simulink model "AUV_Multi_MPC"  (R2023a)
settings: Solver=ode23t  StartTime=0.0  StopTime=300  MaxStep=0.01  RelTol=1e-3  EnableMultiTasking=on
PreLoadFcn:
  | AUV_VehicleParameters;
  | Vehicle.Body.markeropacity = 0;
InitFcn:
  | %% ========================= SAMPLE TIME =========================
  | Ts = 0.1;
  | %% ========================= MPC: SURGE X =========================
  | nx = 1; nu = 1; ny = 1;
  | 
  | A = 0.9; B = 0.1; C = 1; D = 0;
  | plant = ss(A, B, C, D, Ts);
  | mpc1 = mpc(plant, Ts);
  | 
  | % Cấu hình như bình thường
  | mpc1.PredictionHorizon = 10;
  | mpc1.ControlHorizon = 2;
  | 
  | mpc1.Weights.OV = 7.5; % đủ mạnh để bám
  | mpc1.Weights.MV = 0.08; % cho dùng lực nhiều hơn
  | mpc1.Weights.MVRate = 0.25; % vừa mượt vừa linh hoạt
  | mpc1.MV.Min = -40;
  | mpc1.MV.Max = 40;
  | mpc1.OV.Min = 0;
  | mpc1.OV.Max = 2;
  | 
  | % Ràng buộc về thay đổi lực
  | mpc1.MV.RateMin = -12.5;
  | mpc1.MV.RateMax = 12.5;
  | %% ========================= MPC OUTER LOOP FOR DEPTH (Z) =========================
  | % ===== Baseline outer MPC for depth =====
  | u0 = 1.2;
  | 
  | A = 1;
  | B = -Ts*u0;
  | C = 1;
  | D = 0;
  | 
  | plant_z = ss(A,B,C,D,Ts);
  | 
  | mpc_z = mpc(plant_z,Ts);
  | mpc_z.PredictionHorizon = 10;
  | mpc_z.ControlHorizon    = 2;
  | 
  | mpc_z.Weights.OV     = 12;
  | mpc_z.Weights.MV     = 0.01;
  | mpc_z.Weights.MVRate = 0.1;
  | 
  | theta_ref_max = deg2rad(18);
  | mpc_z.MV.Min = -theta_ref_max;
  | mpc_z.MV.Max =  theta_ref_max;
  | 
  | mpc_z.MV.RateMin = -deg2rad(4);
  | mpc_z.MV.RateMax =  deg2rad(4);
  | 
  | 
  | %% ========================= MPC OUTER LOOP FOR HEADING =========================
  | A = 1;
  | B = Ts;
  | C = 1;
  | D = 0;
  | 
  | plant_psi = ss(A,B,C,D,Ts);
  | mpc_psi = mpc(plant_psi,Ts);
  | 
  | ... (+13 lines)
StopFcn:
  | try
  |     S = out;
  | 
  |     % ===============================
  |     % CHỌN HỆ QUY CHIẾU
  |     % ===============================
  |     USE_UP = true;   % true = ENU (Up), false = NED (Down)
  | 
  |     % ===============================
  |     % AUV position (NED gốc)
  |     % ===============================
  |     P  = squeeze(S.auv_position.signals.values);   % [Xn Ye Zd]
  |     tP = S.auv_position.time(:);
  | 
  |     Xn = P(:,1);   % North
  |     Ye = P(:,2);   % East
  |     Zd = P(:,3);   % Down (+)
  | 
  |     % ===============================
  |     % Reference vector
  |     % ===============================
  |     R = squeeze(S.auv_reference.signals.values);  % [V D psi]
  |     t = S.auv_reference.time(:);
  | 
  |     V   = R(:,1);      % speed
  |     D   = R(:,2);      % depth (Down +)
  |     psi = R(:,3);      % heading (rad)
  | 
  |     % ===============================
  |     % Reconstruct reference trajectory (NED)
  |     % ===============================
  |     Xr = Xn(1) + cumtrapz(t, V .* cos(psi));   % North
  |     Yr = Ye(1) + cumtrapz(t, V .* sin(psi));   % East
  |     Zr_down = Zd(1) + (D - D(1));              % Down (+)
  | 
  |     % ===============================
  |     % CHUYỂN HỆ (nếu cần)
  |     % ===============================
  |     if USE_UP
  |         Za  = -Zd;        % Up
  |         Zr  = -Zr_down;   % Up
  |         zlbl = 'Z (Up, m)';
  |     else
  |         Za  = Zd;         % Down
  |         Zr  = Zr_down;
  |         zlbl = 'Z (Down, m)';
  |     end
  | 
  |     % ===============================
  |     % Plot
  |     % ===============================
  |     f = figure(2); clf(f);
  |     set(f,'Name','AUV vs Reference','NumberTitle','off');
  | 
  |     ax = gca;
  |     ax.SortMethod = 'childorder';
  | 
  |     hRef   = plot3(Xr, Yr, Zr, '--', ...
  |                    'Color',[0.6 0.6 0.6], 'LineWidth',1.2);
  |     hold on
  | ... (+24 lines)
model workspace: external: MATLAB File AUV_DataFile_ORIG.m (data not in the file)
undefined symbols (not defined in the file): Environment, Multibody, Newton, Raphson, smiData, X, x, Y, y, Z
libraries: sm_lib x3123, nesl_utility x51, sharedutil x8, simulink x6, AUVCustomPrimitives_Lib x4, mpclib x3, fuzblock x2, instrumentseriallib x2, shared6dof x1, slpidlib x1, aerolibasang x1, aerolibadyn x1
(part 2 of 72)

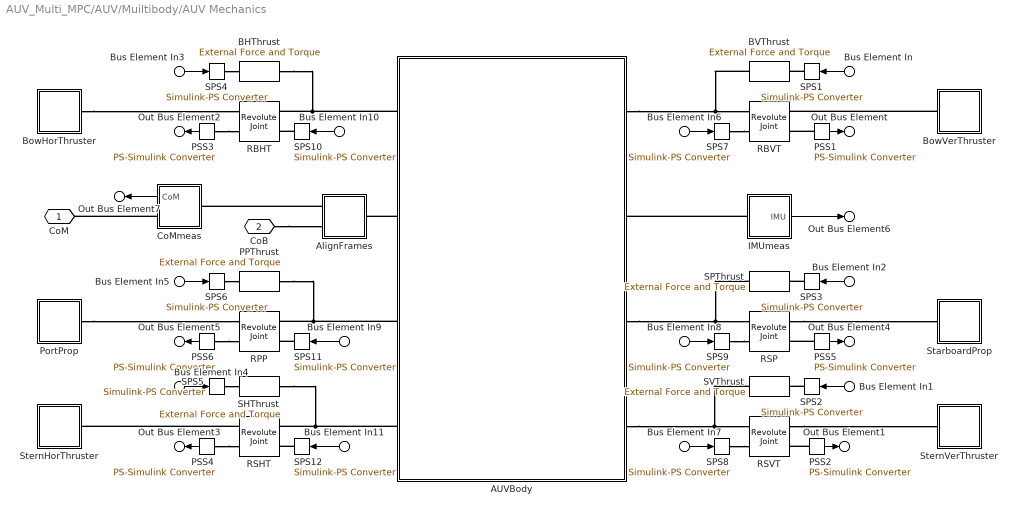
== system AUV_Multi_MPC/AUV/Muiltibody/AUV Mechanics ==
  Bus Element In : Inport  PortName=Actuators  Element=Thrusters.BVTf
  Bus Element In1 : Inport  PortName=Actuators  Element=Thrusters.SVTf
  Bus Element In3 : Inport  PortName=Actuators  Element=Thrusters.BHTf
  Bus Element In4 : Inport  PortName=Actuators  Element=Thrusters.SHTf
  Bus Element In6 : Inport  PortName=Actuators  Element=Thrusters.BVTt
  Bus Element In7 : Inport  PortName=Actuators  Element=Thrusters.SVTt
  Bus Element In10 : Inport  PortName=Actuators  Element=Thrusters.BHTt
  Bus Element In11 : Inport  PortName=Actuators  Element=Thrusters.SHTt
  Bus Element In2 : Inport  PortName=Actuators  Element=Propellers.SPf
  Bus Element In5 : Inport  PortName=Actuators  Element=Propellers.PPf
  Bus Element In8 : Inport  PortName=Actuators  Element=Propellers.SPt
  Bus Element In9 : Inport  PortName=Actuators  Element=Propellers.PPt
  AUVBody : Subsystem
      mask Display: image('AUVBody.png');
  AlignFrames : Subsystem
  BHThrust : sm_lib/Forces and Torques/External Force and Torque  ForceResolutionFrame=AttachedFrame  EnableForceX=off  EnableForceY=off  EnableForceZ=on  EnableForce=off  TorqueResolutionFrame=AttachedFrame  EnableTorqueX=off  EnableTorqueY=off  EnableTorqueZ=off  EnableTorque=off
  BVThrust : sm_lib/Forces and Torques/External Force and Torque  ForceResolutionFrame=AttachedFrame  EnableForceX=off  EnableForceY=off  EnableForceZ=on  EnableForce=off  TorqueResolutionFrame=AttachedFrame  EnableTorqueX=off  EnableTorqueY=off  EnableTorqueZ=off  EnableTorque=off
  BowHorThruster : Subsystem
      mask Display: image('TunnelThrusterProp.png',[0.15,0.25,0.7,0.5]);
  BowVerThruster : Subsystem
      mask Display: image('TunnelThrusterProp.png',[0.15,0.25,0.7,0.5]);
  CoMmeas : Subsystem
  IMUmeas : Subsystem
  PPThrust : sm_lib/Forces and Torques/External Force and Torque  ForceResolutionFrame=AttachedFrame  EnableForceX=off  EnableForceY=off  EnableForceZ=on  EnableForce=off  TorqueResolutionFrame=AttachedFrame  EnableTorqueX=off  EnableTorqueY=off  EnableTorqueZ=off  EnableTorque=off
  PSS{1..6} (6 alike) : nesl_utility/PS-Simulink Converter  PhysicalDomain=network_engine_domain  SubClassName=ps_output  LeftPortType=input  RightPortType=output  PseudoPeriodic=off  Frequencies=[]  VectorFormat=1-D array  Unit=rad/s  AffineConversion=off
  PortProp : Subsystem
      mask Display: image('MainProp.png',[0.1,0.1,0.8,0.8]);
  RBHT : sm_lib/Joints/Revolute Joint  JointMode=Normal  SenseConstraintForce=off  SenseConstraintForceX=off  SenseConstraintForceY=off  SenseConstraintForceZ=off  SenseConstraintTorque=off  SenseConstraintTorqueX=off  SenseConstraintTorqueY=off  SenseConstraintTorqueZ=off  SenseTotalForce=off  SenseTotalForceX=off  SenseTotalForceY=off  SenseTotalForceZ=off  SenseTotalTorque=off  SenseTotalTorqueX=off  SenseTotalTorqueY=off  SenseTotalTorqueZ=off  CompositeWrenchDir=FollowerOnBase  CompositeWrenchFrame=BaseFrame  EquilibriumPosition=0  EquilibriumPositionUnits=rad  SpringStiffness=0  SpringStiffnessUnits=N*m/rad  DampingCoefficient=0  DampingCoefficientUnits=N*m/(rad/s)  TorqueActuationMode=InputTorque  MotionActuationMode=ComputedMotion  SensePosition=off  SenseVelocity=on  SenseAcceleration=off  SenseTorqueForce=off  SenseLowerLimitTorqueForce=off  SenseUpperLimitTorqueForce=off  LowerLimitSpecify=off  LowerLimitBound=-90  LowerLimitBoundUnits=deg  LowerLimitStiffness=1e4  LowerLimitStiffnessUnits=N*m/deg  LowerLimitDamping=10  LowerLimitDampingUnits=N*m/(deg/s)  LowerLimitTransitionRegionWidth=0.1  LowerLimitTransitionRegionWidthUnits=deg  UpperLimitSpecify=off  UpperLimitBound=90  UpperLimitBoundUnits=deg  UpperLimitStiffness=1e4  UpperLimitStiffnessUnits=N*m/deg  UpperLimitDamping=10  UpperLimitDampingUnits=N*m/(deg/s)  UpperLimitTransitionRegionWidth=0.1  UpperLimitTransitionRegionWidthUnits=deg  PositionTargetSpecify=on  PositionTargetPriority=Low  PositionTargetValue=smiData.RevoluteJoint(5).Rz.Pos  PositionTargetValueUnits=deg  VelocityTargetSpecify=off  VelocityTargetPriority=High  VelocityTargetValue=0  VelocityTargetValueUnits=deg/s
  RBVT : sm_lib/Joints/Revolute Joint  JointMode=Normal  SenseConstraintForce=off  SenseConstraintForceX=off  SenseConstraintForceY=off  SenseConstraintForceZ=off  SenseConstraintTorque=off  SenseConstraintTorqueX=off  SenseConstraintTorqueY=off  SenseConstraintTorqueZ=off  SenseTotalForce=off  SenseTotalForceX=off  SenseTotalForceY=off  SenseTotalForceZ=off  SenseTotalTorque=off  SenseTotalTorqueX=off  SenseTotalTorqueY=off  SenseTotalTorqueZ=off  CompositeWrenchDir=FollowerOnBase  CompositeWrenchFrame=BaseFrame  EquilibriumPosition=0  EquilibriumPositionUnits=rad  SpringStiffness=0  SpringStiffnessUnits=N*m/rad  DampingCoefficient=0  DampingCoefficientUnits=N*m/(rad/s)  TorqueActuationMode=InputTorque  MotionActuationMode=ComputedMotion  SensePosition=off  SenseVelocity=on  SenseAcceleration=off  SenseTorqueForce=off  SenseLowerLimitTorqueForce=off  SenseUpperLimitTorqueForce=off  LowerLimitSpecify=off  LowerLimitBound=-90  LowerLimitBoundUnits=deg  LowerLimitStiffness=1e4  LowerLimitStiffnessUnits=N*m/deg  LowerLimitDamping=10  LowerLimitDampingUnits=N*m/(deg/s)  LowerLimitTransitionRegionWidth=0.1  LowerLimitTransitionRegionWidthUnits=deg  UpperLimitSpecify=off  UpperLimitBound=90  UpperLimitBoundUnits=deg  UpperLimitStiffness=1e4  UpperLimitStiffnessUnits=N*m/deg  UpperLimitDamping=10  UpperLimitDampingUnits=N*m/(deg/s)  UpperLimitTransitionRegionWidth=0.1  UpperLimitTransitionRegionWidthUnits=deg  PositionTargetSpecify=on  PositionTargetPriority=Low  PositionTargetValue=smiData.RevoluteJoint(2).Rz.Pos  PositionTargetValueUnits=deg  VelocityTargetSpecify=off  VelocityTargetPriority=High  VelocityTargetValue=0  VelocityTargetValueUnits=deg/s
  RPP : sm_lib/Joints/Revolute Joint  JointMode=Normal  SenseConstraintForce=off  SenseConstraintForceX=off  SenseConstraintForceY=off  SenseConstraintForceZ=off  SenseConstraintTorque=off  SenseConstraintTorqueX=off  SenseConstraintTorqueY=off  SenseConstraintTorqueZ=off  SenseTotalForce=off  SenseTotalForceX=off  SenseTotalForceY=off  SenseTotalForceZ=off  SenseTotalTorque=off  SenseTotalTorqueX=off  SenseTotalTorqueY=off  SenseTotalTorqueZ=off  CompositeWrenchDir=FollowerOnBase  CompositeWrenchFrame=BaseFrame  EquilibriumPosition=0  EquilibriumPositionUnits=rad  SpringStiffness=0  SpringStiffnessUnits=N*m/rad  DampingCoefficient=0  DampingCoefficientUnits=N*m/(rad/s)  TorqueActuationMode=InputTorque  MotionActuationMode=ComputedMotion  SensePosition=off  SenseVelocity=on  SenseAcceleration=off  SenseTorqueForce=off  SenseLowerLimitTorqueForce=off  SenseUpperLimitTorqueForce=off  LowerLimitSpecify=off  LowerLimitBound=-90  LowerLimitBoundUnits=deg  LowerLimitStiffness=1e4  LowerLimitStiffnessUnits=N*m/deg  LowerLimitDamping=10  LowerLimitDampingUnits=N*m/(deg/s)  LowerLimitTransitionRegionWidth=0.1  LowerLimitTransitionRegionWidthUnits=deg  UpperLimitSpecify=off  UpperLimitBound=90  UpperLimitBoundUnits=deg  UpperLimitStiffness=1e4  UpperLimitStiffnessUnits=N*m/deg  UpperLimitDamping=10  UpperLimitDampingUnits=N*m/(deg/s)  UpperLimitTransitionRegionWidth=0.1  UpperLimitTransitionRegionWidthUnits=deg  PositionTargetSpecify=on  PositionTargetPriority=Low  PositionTargetValue=smiData.RevoluteJoint(4).Rz.Pos  PositionTargetValueUnits=deg  VelocityTargetSpecify=off  VelocityTargetPriority=High  VelocityTargetValue=0  VelocityTargetValueUnits=deg/s
  RSHT : sm_lib/Joints/Revolute Joint  JointMode=Normal  SenseConstraintForce=off  SenseConstraintForceX=off  SenseConstraintForceY=off  SenseConstraintForceZ=off  SenseConstraintTorque=off  SenseConstraintTorqueX=off  SenseConstraintTorqueY=off  SenseConstraintTorqueZ=off  SenseTotalForce=off  SenseTotalForceX=off  SenseTotalForceY=off  SenseTotalForceZ=off  SenseTotalTorque=off  SenseTotalTorqueX=off  SenseTotalTorqueY=off  SenseTotalTorqueZ=off  CompositeWrenchDir=FollowerOnBase  CompositeWrenchFrame=BaseFrame  EquilibriumPosition=0  EquilibriumPositionUnits=rad  SpringStiffness=0  SpringStiffnessUnits=N*m/rad  DampingCoefficient=0  DampingCoefficientUnits=N*m/(rad/s)  TorqueActuationMode=InputTorque  MotionActuationMode=ComputedMotion  SensePosition=off  SenseVelocity=on  SenseAcceleration=off  SenseTorqueForce=off  SenseLowerLimitTorqueForce=off  SenseUpperLimitTorqueForce=off  LowerLimitSpecify=off  LowerLimitBound=-90  LowerLimitBoundUnits=deg  LowerLimitStiffness=1e4  LowerLimitStiffnessUnits=N*m/deg  LowerLimitDamping=10  LowerLimitDampingUnits=N*m/(deg/s)  LowerLimitTransitionRegionWidth=0.1  LowerLimitTransitionRegionWidthUnits=deg  UpperLimitSpecify=off  UpperLimitBound=90  UpperLimitBoundUnits=deg  UpperLimitStiffness=1e4  UpperLimitStiffnessUnits=N*m/deg  UpperLimitDamping=10  UpperLimitDampingUnits=N*m/(deg/s)  UpperLimitTransitionRegionWidth=0.1  UpperLimitTransitionRegionWidthUnits=deg  PositionTargetSpecify=on  PositionTargetPriority=Low  PositionTargetValue=smiData.RevoluteJoint(6).Rz.Pos  PositionTargetValueUnits=deg  VelocityTargetSpecify=off  VelocityTargetPriority=High  VelocityTargetValue=0  VelocityTargetValueUnits=deg/s
  RSP : sm_lib/Joints/Revolute Joint  JointMode=Normal  SenseConstraintForce=off  SenseConstraintForceX=off  SenseConstraintForceY=off  SenseConstraintForceZ=off  SenseConstraintTorque=off  SenseConstraintTorqueX=off  SenseConstraintTorqueY=off  SenseConstraintTorqueZ=off  SenseTotalForce=off  SenseTotalForceX=off  SenseTotalForceY=off  SenseTotalForceZ=off  SenseTotalTorque=off  SenseTotalTorqueX=off  SenseTotalTorqueY=off  SenseTotalTorqueZ=off  CompositeWrenchDir=FollowerOnBase  CompositeWrenchFrame=BaseFrame  EquilibriumPosition=0  EquilibriumPositionUnits=rad  SpringStiffness=0  SpringStiffnessUnits=N*m/rad  DampingCoefficient=0  DampingCoefficientUnits=N*m/(rad/s)  TorqueActuationMode=InputTorque  MotionActuationMode=ComputedMotion  SensePosition=off  SenseVelocity=on  SenseAcceleration=off  SenseTorqueForce=off  SenseLowerLimitTorqueForce=off  SenseUpperLimitTorqueForce=off  LowerLimitSpecify=off  LowerLimitBound=-90  LowerLimitBoundUnits=deg  LowerLimitStiffness=1e4  LowerLimitStiffnessUnits=N*m/deg  LowerLimitDamping=10  LowerLimitDampingUnits=N*m/(deg/s)  LowerLimitTransitionRegionWidth=0.1  LowerLimitTransitionRegionWidthUnits=deg  UpperLimitSpecify=off  UpperLimitBound=90  UpperLimitBoundUnits=deg  UpperLimitStiffness=1e4  UpperLimitStiffnessUnits=N*m/deg  UpperLimitDamping=10  UpperLimitDampingUnits=N*m/(deg/s)  UpperLimitTransitionRegionWidth=0.1  UpperLimitTransitionRegionWidthUnits=deg  PositionTargetSpecify=on  PositionTargetPriority=Low  PositionTargetValue=smiData.RevoluteJoint(1).Rz.Pos  PositionTargetValueUnits=deg  VelocityTargetSpecify=off  VelocityTargetPriority=High  VelocityTargetValue=0  VelocityTargetValueUnits=deg/s
  RSVT : sm_lib/Joints/Revolute Joint  JointMode=Normal  SenseConstraintForce=off  SenseConstraintForceX=off  SenseConstraintForceY=off  SenseConstraintForceZ=off  SenseConstraintTorque=off  SenseConstraintTorqueX=off  SenseConstraintTorqueY=off  SenseConstraintTorqueZ=off  SenseTotalForce=off  SenseTotalForceX=off  SenseTotalForceY=off  SenseTotalForceZ=off  SenseTotalTorque=off  SenseTotalTorqueX=off  SenseTotalTorqueY=off  SenseTotalTorqueZ=off  CompositeWrenchDir=FollowerOnBase  CompositeWrenchFrame=BaseFrame  EquilibriumPosition=0  EquilibriumPositionUnits=rad  SpringStiffness=0  SpringStiffnessUnits=N*m/rad  DampingCoefficient=0  DampingCoefficientUnits=N*m/(rad/s)  TorqueActuationMode=InputTorque  MotionActuationMode=ComputedMotion  SensePosition=off  SenseVelocity=on  SenseAcceleration=off  SenseTorqueForce=off  SenseLowerLimitTorqueForce=off  SenseUpperLimitTorqueForce=off  LowerLimitSpecify=off  LowerLimitBound=-90  LowerLimitBoundUnits=deg  LowerLimitStiffness=1e4  LowerLimitStiffnessUnits=N*m/deg  LowerLimitDamping=10  LowerLimitDampingUnits=N*m/(deg/s)  LowerLimitTransitionRegionWidth=0.1  LowerLimitTransitionRegionWidthUnits=deg  UpperLimitSpecify=off  UpperLimitBound=90  UpperLimitBoundUnits=deg  UpperLimitStiffness=1e4  UpperLimitStiffnessUnits=N*m/deg  UpperLimitDamping=10  UpperLimitDampingUnits=N*m/(deg/s)  UpperLimitTransitionRegionWidth=0.1  UpperLimitTransitionRegionWidthUnits=deg  PositionTargetSpecify=on  PositionTargetPriority=Low  PositionTargetValue=smiData.RevoluteJoint(3).Rz.Pos  PositionTargetValueUnits=deg  VelocityTargetSpecify=off  VelocityTargetPriority=High  VelocityTargetValue=0  VelocityTargetValueUnits=deg/s
  SHThrust : sm_lib/Forces and Torques/External Force and Torque  ForceResolutionFrame=AttachedFrame  EnableForceX=off  EnableForceY=off  EnableForceZ=on  EnableForce=off  TorqueResolutionFrame=AttachedFrame  EnableTorqueX=off  EnableTorqueY=off  EnableTorqueZ=off  EnableTorque=off
  SPS{1..6} (6 alike) : nesl_utility/Simulink-PS Converter  PhysicalDomain=network_engine_domain  SubClassName=ps_input  LeftPortType=input  RightPortType=output  PseudoPeriodic=off  Frequencies=[]  NoiseDistribution=none  NoiseParameters=[]  Unit=N  AffineConversion=off  FilteringAndDerivatives=provide  SimscapeFilterOrder=1  InputFilterTimeConstant=0.001  UdotUserProvided=0
  SPS{7..12} (6 alike) : nesl_utility/Simulink-PS Converter  PhysicalDomain=network_engine_domain  SubClassName=ps_input  LeftPortType=input  RightPortType=output  PseudoPeriodic=off  Frequencies=[]  NoiseDistribution=none  NoiseParameters=[]  Unit=N*m  AffineConversion=off  FilteringAndDerivatives=provide  SimscapeFilterOrder=1  InputFilterTimeConstant=0.001  UdotUserProvided=0
  SPThrust : sm_lib/Forces and Torques/External Force and Torque  ForceResolutionFrame=AttachedFrame  EnableForceX=off  EnableForceY=off  EnableForceZ=on  EnableForce=off  TorqueResolutionFrame=AttachedFrame  EnableTorqueX=off  EnableTorqueY=off  EnableTorqueZ=off  EnableTorque=off
  SVThrust : sm_lib/Forces and Torques/External Force and Torque  ForceResolutionFrame=AttachedFrame  EnableForceX=off  EnableForceY=off  EnableForceZ=on  EnableForce=off  TorqueResolutionFrame=AttachedFrame  EnableTorqueX=off  EnableTorqueY=off  EnableTorqueZ=off  EnableTorque=off
  StarboardProp : Subsystem
      mask Display: image('MainProp.png',[0.1,0.1,0.8,0.8]);
  SternHorThruster : Subsystem
      mask Display: image('TunnelThrusterProp.png',[0.15,0.25,0.7,0.5]);
  SternVerThruster : Subsystem
      mask Display: image('TunnelThrusterProp.png',[0.15,0.25,0.7,0.5]);
  CoM : PMIOPort  Side=Left
  CoB : PMIOPort  Port=2  Side=Left
  Out Bus Element6 : Outport  PortName=Vehicle  Element=IMU
  Out Bus Element4 : Outport  PortName=Vehicle  Element=Propellers.SPw
  Out Bus Element5 : Outport  PortName=Vehicle  Element=Propellers.PPw
  Out Bus Element : Outport  PortName=Vehicle  Element=Thrusters.BVTw
  Out Bus Element1 : Outport  PortName=Vehicle  Element=Thrusters.SVTw
  Out Bus Element2 : Outport  PortName=Vehicle  Element=Thrusters.BHTw
  Out Bus Element3 : Outport  PortName=Vehicle  Element=Thrusters.SHTw
  Out Bus Element7 : Outport  PortName=Vehicle  Element=CoM
  wires:
  PSS1/1 -> Out Bus Element/1
  PSS2/1 -> Out Bus Element1/1
  PSS3/1 -> Out Bus Element2/1
  PSS4/1 -> Out Bus Element3/1
  PSS5/1 -> Out Bus Element4/1
  PSS6/1 -> Out Bus Element5/1
  IMUmeas/1(IMU) -> Out Bus Element6/1
  Bus Element In/1 -> SPS1/1
  Bus Element In1/1 -> SPS2/1
  Bus Element In2/1 -> SPS3/1
  Bus Element In3/1 -> SPS4/1
  Bus Element In4/1 -> SPS5/1
  Bus Element In5/1 -> SPS6/1
  CoMmeas/1(CoM) -> Out Bus Element7/1
  Bus Element In6/1 -> SPS7/1
  Bus Element In7/1 -> SPS8/1
  Bus Element In8/1 -> SPS9/1
  Bus Element In9/1 -> SPS11/1
  Bus Element In10/1 -> SPS10/1
  Bus Element In11/1 -> SPS12/1
  connections:
  PortProp/LConn1 -- RPP/RConn1
  AUVBody/LConn1 -- BHThrust/RConn1 -- RBHT/LConn1
  AUVBody/LConn4 -- SHThrust/RConn1 -- RSHT/LConn1
  BowVerThruster/LConn1 -- RBVT/RConn1
  RSP/RConn1 -- StarboardProp/LConn1
  AUVBody/RConn4 -- RSVT/LConn1 -- SVThrust/RConn1
  BowHorThruster/LConn1 -- RBHT/RConn1
  RSVT/RConn1 -- SternVerThruster/LConn1
  AUVBody/RConn1 -- RBVT/LConn1 -- BVThrust/RConn1
  AUVBody/RConn3 -- RSP/LConn1 -- SPThrust/RConn1
  RSHT/RConn1 -- SternHorThruster/LConn1
  AUVBody/LConn3 -- PPThrust/RConn1 -- RPP/LConn1
  AUVBody/LConn2 -- AlignFrames/RConn1
  PSS1/LConn1 -- RBVT/RConn2
  PSS2/LConn1 -- RSVT/RConn2
  PSS3/LConn1 -- RBHT/RConn2
  PSS4/LConn1 -- RSHT/RConn2
  PSS5/LConn1 -- RSP/RConn2
  PSS6/LConn1 -- RPP/RConn2
  IMUmeas/LConn1 -- AUVBody/RConn2
  SPS1/RConn1 -- BVThrust/LConn1
  SPS2/RConn1 -- SVThrust/LConn1
  SPS3/RConn1 -- SPThrust/LConn1
  SPS4/RConn1 -- BHThrust/LConn1
  SPS5/RConn1 -- SHThrust/LConn1
  SPS6/RConn1 -- PPThrust/LConn1
  AlignFrames/LConn1 -- CoMmeas/LConn1
  CoMmeas/RConn1 -- CoM/RConn1
  SPS7/RConn1 -- RBVT/LConn2
  SPS8/RConn1 -- RSVT/LConn2
  SPS9/RConn1 -- RSP/LConn2
  SPS10/RConn1 -- RBHT/LConn2
  SPS11/RConn1 -- RPP/LConn2
  SPS12/RConn1 -- RSHT/LConn2
  CoB/RConn1 -- AlignFrames/LConn2

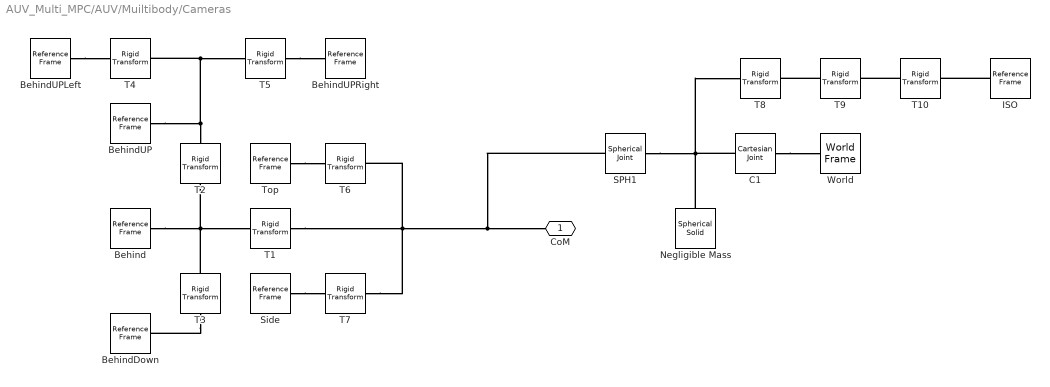
== system AUV_Multi_MPC/AUV/Muiltibody/Cameras ==
  Behind : sm_lib/Frames and Transforms/Reference Frame
  BehindDown : sm_lib/Frames and Transforms/Reference Frame
  BehindUP : sm_lib/Frames and Transforms/Reference Frame
  BehindUPLeft : sm_lib/Frames and Transforms/Reference Frame
  BehindUPRight : sm_lib/Frames and Transforms/Reference Frame
  C1 : sm_lib/Joints/Cartesian Joint  JointMode=Normal  SenseConstraintForce=off  SenseConstraintForceX=off  SenseConstraintForceY=off  SenseConstraintForceZ=off  SenseConstraintTorque=off  SenseConstraintTorqueX=off  SenseConstraintTorqueY=off  SenseConstraintTorqueZ=off  SenseTotalForce=off  SenseTotalForceX=off  SenseTotalForceY=off  SenseTotalForceZ=off  SenseTotalTorque=off  SenseTotalTorqueX=off  SenseTotalTorqueY=off  SenseTotalTorqueZ=off  CompositeWrenchDir=FollowerOnBase  CompositeWrenchFrame=BaseFrame  PxEquilibriumPosition=0  PxEquilibriumPositionUnits=m  PxSpringStiffness=0  PxSpringStiffnessUnits=N/m  PxDampingCoefficient=0  PxDampingCoefficientUnits=N/(m/s)  PxTorqueActuationMode=NoTorque  PxMotionActuationMode=ComputedMotion  PxSensePosition=off  PxSenseVelocity=off  PxSenseAcceleration=off  PxSenseTorqueForce=off  PxSenseLowerLimitTorqueForce=off  PxSenseUpperLimitTorqueForce=off  PxLowerLimitSpecify=off  PxLowerLimitBound=-1  PxLowerLimitBoundUnits=m  PxLowerLimitStiffness=1e6  PxLowerLimitStiffnessUnits=N/m  PxLowerLimitDamping=1e3  PxLowerLimitDampingUnits=N/(m/s)  PxLowerLimitTransitionRegionWidth=1e-4  PxLowerLimitTransitionRegionWidthUnits=m  PxUpperLimitSpecify=off  PxUpperLimitBound=1  PxUpperLimitBoundUnits=m  PxUpperLimitStiffness=1e6  PxUpperLimitStiffnessUnits=N/m  PxUpperLimitDamping=1e3  PxUpperLimitDampingUnits=N/(m/s)  PxUpperLimitTransitionRegionWidth=1e-4  PxUpperLimitTransitionRegionWidthUnits=m  PxPositionTargetSpecify=off  PxPositionTargetPriority=High  PxPositionTargetValue=0  PxPositionTargetValueUnits=m  PxVelocityTargetSpecify=off  PxVelocityTargetPriority=High  PxVelocityTargetValue=0  PxVelocityTargetValueUnits=m/s  PyEquilibriumPosition=0  PyEquilibriumPositionUnits=m  PySpringStiffness=0  PySpringStiffnessUnits=N/m  PyDampingCoefficient=0  PyDampingCoefficientUnits=N/(m/s)  PyTorqueActuationMode=NoTorque  PyMotionActuationMode=ComputedMotion  PySensePosition=off  PySenseVelocity=off  PySenseAcceleration=off  PySenseTorqueForce=off  PySenseLowerLimitTorqueForce=off  PySenseUpperLimitTorqueForce=off  PyLowerLimitSpecify=off  PyLowerLimitBound=-1  PyLowerLimitBoundUnits=m  PyLowerLimitStiffness=1e6  PyLowerLimitStiffnessUnits=N/m  PyLowerLimitDamping=1e3  PyLowerLimitDampingUnits=N/(m/s)  PyLowerLimitTransitionRegionWidth=1e-4  PyLowerLimitTransitionRegionWidthUnits=m  PyUpperLimitSpecify=off  PyUpperLimitBound=1  PyUpperLimitBoundUnits=m  PyUpperLimitStiffness=1e6  PyUpperLimitStiffnessUnits=N/m  PyUpperLimitDamping=1e3  PyUpperLimitDampingUnits=N/(m/s)  PyUpperLimitTransitionRegionWidth=1e-4  PyUpperLimitTransitionRegionWidthUnits=m  PyPositionTargetSpecify=off  PyPositionTargetPriority=High  PyPositionTargetValue=0  PyPositionTargetValueUnits=m  PyVelocityTargetSpecify=off  PyVelocityTargetPriority=High  PyVelocityTargetValue=0  PyVelocityTargetValueUnits=m/s  PzEquilibriumPosition=0  PzEquilibriumPositionUnits=m  PzSpringStiffness=0  PzSpringStiffnessUnits=N/m  PzDampingCoefficient=0  PzDampingCoefficientUnits=N/(m/s)  PzTorqueActuationMode=NoTorque  PzMotionActuationMode=ComputedMotion  PzSensePosition=off  PzSenseVelocity=off  PzSenseAcceleration=off  PzSenseTorqueForce=off  PzSenseLowerLimitTorqueForce=off  PzSenseUpperLimitTorqueForce=off  PzLowerLimitSpecify=off  PzLowerLimitBound=-1  PzLowerLimitBoundUnits=m  PzLowerLimitStiffness=1e6  PzLowerLimitStiffnessUnits=N/m  PzLowerLimitDamping=1e3  PzLowerLimitDampingUnits=N/(m/s)  PzLowerLimitTransitionRegionWidth=1e-4  PzLowerLimitTransitionRegionWidthUnits=m  PzUpperLimitSpecify=off  PzUpperLimitBound=1  PzUpperLimitBoundUnits=m  PzUpperLimitStiffness=1e6  PzUpperLimitStiffnessUnits=N/m  PzUpperLimitDamping=1e3  PzUpperLimitDampingUnits=N/(m/s)  PzUpperLimitTransitionRegionWidth=1e-4  PzUpperLimitTransitionRegionWidthUnits=m  PzPositionTargetSpecify=off  PzPositionTargetPriority=High  PzPositionTargetValue=0  PzPositionTargetValueUnits=m  PzVelocityTargetSpecify=off  PzVelocityTargetPriority=High  PzVelocityTargetValue=0  PzVelocityTargetValueUnits=m/s
  ISO : sm_lib/Frames and Transforms/Reference Frame
  Negligible Mass : sm_lib/Body Elements/Spherical Solid  GraphicAmbientColor=[0.15 0.15 0.15 1.0]  BasedOnType=Mass  CenterOfMass=[0 0 0]  CenterOfMassUnits=m  GraphicDiffuseColor=[0.5 0.5 0.5]  Density=1000  DensityUnits=kg/m^3  DoExposeReferenceFrame=on  GraphicEmissiveColor=[0.0 0.0 0.0 1.0]  ExportEntireGeometry=off  SerializedExposedGeometries=<ExposedGeometries/>  SerializedFrames=<Frames/>  MarkerShape=Sphere  MarkerSize=10  GraphicType=FromGeometry  InertiaType=CalculateFromGeometry  Mass=1e-6  MassUnits=kg  MomentsOfInertia=[1 1 1]  MomentsOfInertiaUnits=kg*m^2  GraphicOpacity=0  ProductsOfInertia=[0 0 0]  ProductsOfInertiaUnits=kg*m^2  GraphicShininess=75  GraphicSpecularColor=[0.5 0.5 0.5 1.0]  SphereRadius=1e-3  SphereRadiusUnits=m  GraphicVisPropType=SimpleVisualProperties
  SPH1 : sm_lib/Joints/Spherical Joint  JointMode=Normal  SenseConstraintForce=off  SenseConstraintForceX=off  SenseConstraintForceY=off  SenseConstraintForceZ=off  SenseConstraintTorque=off  SenseConstraintTorqueX=off  SenseConstraintTorqueY=off  SenseConstraintTorqueZ=off  SenseTotalForce=off  SenseTotalForceX=off  SenseTotalForceY=off  SenseTotalForceZ=off  SenseTotalTorque=off  SenseTotalTorqueX=off  SenseTotalTorqueY=off  SenseTotalTorqueZ=off  CompositeWrenchDir=FollowerOnBase  CompositeWrenchFrame=BaseFrame  EqPosRotationMethod=None  EqPosRotationAngleUnits=deg  EqPosRotationStandardAxis=+Z  EqPosRotationAngle=0.0  EqPosRotationArbitraryAxis=[0 0 1]  EqPosFollAlignAxisA=+X  EqPosBaseAlignAxisA=+Y  EqPosFollAlignAxisB=+Y  EqPosBaseAlignAxisB=+Z  EqPosRotationSequenceAxes=FollowerAxes  EqPosRotationSequence=XYX  EqPosRotationSequenceAngles=[0 0 0]  EqPosRotationSequenceAnglesUnits=deg  EqPosRotationMatrix=[1 0 0; 0 1 0; 0 0 1]  EqPosQuaternion=[1 0 0 0]  SpringStiffness=0  SpringStiffnessUnits=N*m/deg  DampingCoefficient=0  DampingCoefficientUnits=N*m/(deg/s)  ActuateTorqueX=off  ActuateTorqueY=off  ActuateTorqueZ=off  ActuateTorque=off  TorqueActuationMode=NoTorque  MotionActuationMode=ComputedMotion  ActuationFrame=BaseFrame  SensePosition=off  SenseVelocityX=off  SenseVelocityY=off  SenseVelocityZ=off  SenseVelocity=off  SenseAccelerationX=off  SenseAccelerationY=off  SenseAccelerationZ=off  SenseAcceleration=off  SenseTorqueX=off  SenseTorqueY=off  SenseTorqueZ=off  SenseTorqueForce=off  SenseLowerLimitTorqueMag=off  SenseUpperLimitTorqueMag=off  SensingFrame=BaseFrame  LowerLimitSpecify=off  LowerLimitBound=15  LowerLimitBoundUnits=deg  LowerLimitStiffness=1e4  LowerLimitStiffnessUnits=N*m/deg  LowerLimitDamping=10  LowerLimitDampingUnits=N*m/(deg/s)  LowerLimitTransitionRegionWidth=0.1  LowerLimitTransitionRegionWidthUnits=deg  UpperLimitSpecify=off  UpperLimitBound=45  UpperLimitBoundUnits=deg  UpperLimitStiffness=1e4  UpperLimitStiffnessUnits=N*m/deg  UpperLimitDamping=10  UpperLimitDampingUnits=N*m/(deg/s)  UpperLimitTransitionRegionWidth=0.1  UpperLimitTransitionRegionWidthUnits=deg  PositionTargetRotationMethod=None  PositionTargetRotationAngleUnits=deg  PositionTargetRotationStandardAxis=+Z  PositionTargetRotationAngle=0.0  PositionTargetRotationArbitraryAxis=[0 0 1]  PositionTargetFollAlignAxisA=+X  PositionTargetBaseAlignAxisA=+Y  PositionTargetFollAlignAxisB=+Y  PositionTargetBaseAlignAxisB=+Z  PositionTargetRotationSequenceAxes=FollowerAxes  PositionTargetRotationSequence=XYX  PositionTargetRotationSequenceAngles=[0 0 0]  PositionTargetRotationSequenceAnglesUnits=deg  PositionTargetRotationMatrix=[1 0 0; 0 1 0; 0 0 1]  PositionTargetQuaternion=[1 0 0 0]  PositionTargetSpecify=off  PositionTargetPriority=High  VelocityTargetValue=[0 0 0]  VelocityTargetValueUnits=deg/s  VelocityTargetSpecify=off  VelocityTargetPriority=High  VelocityTargetInFollowerFrame=on
  Side : sm_lib/Frames and Transforms/Reference Frame
  T1 : sm_lib/Frames and Transforms/Rigid Transform  TranslationMethod=Cartesian  TranslationStandardOffset=0  TranslationStandardOffsetUnits=m  TranslationStandardAxis=+Z  TranslationCartesianOffset=[-3 0 0]  TranslationCartesianOffsetUnits=m  TranslationROffset=0  TranslationROffsetUnits=m  TranslationZOffset=0  TranslationZOffsetUnits=m  TranslationThetaOffset=0  TranslationThetaOffsetUnits=deg  RotationMethod=None  RotationAngleUnits=deg  RotationStandardAxis=+Z  RotationAngle=0.0  RotationArbitraryAxis=[0 0 1]  FollAlignAxisA=+X  BaseAlignAxisA=+Y  FollAlignAxisB=+Y  BaseAlignAxisB=+Z  RotationSequenceAxes=FollowerAxes  RotationSequence=XYX  RotationSequenceAngles=[0 0 0]  RotationSequenceAnglesUnits=deg  RotationMatrix=[1 0 0; 0 1 0; 0 0 1]  Quaternion=[1 0 0 0]
  T10 : sm_lib/Frames and Transforms/Rigid Transform  TranslationMethod=Cartesian  TranslationStandardOffset=0  TranslationStandardOffsetUnits=m  TranslationStandardAxis=+Z  TranslationCartesianOffset=[0 -1.5 0]  TranslationCartesianOffsetUnits=m  TranslationROffset=0  TranslationROffsetUnits=m  TranslationZOffset=0  TranslationZOffsetUnits=m  TranslationThetaOffset=0  TranslationThetaOffsetUnits=deg  RotationMethod=None  RotationAngleUnits=deg  RotationStandardAxis=+Z  RotationAngle=0.0  RotationArbitraryAxis=[0 0 1]  FollAlignAxisA=+X  BaseAlignAxisA=+Y  FollAlignAxisB=+Y  BaseAlignAxisB=+Z  RotationSequenceAxes=FollowerAxes  RotationSequence=XYX  RotationSequenceAngles=[0 0 0]  RotationSequenceAnglesUnits=deg  RotationMatrix=[1 0 0; 0 1 0; 0 0 1]  Quaternion=[1 0 0 0]
  T2 : sm_lib/Frames and Transforms/Rigid Transform  TranslationMethod=Cartesian  TranslationStandardOffset=0  TranslationStandardOffsetUnits=m  TranslationStandardAxis=+Z  TranslationCartesianOffset=[0 0 -3]  TranslationCartesianOffsetUnits=m  TranslationROffset=0  TranslationROffsetUnits=m  TranslationZOffset=0  TranslationZOffsetUnits=m  TranslationThetaOffset=0  TranslationThetaOffsetUnits=deg  RotationMethod=None  RotationAngleUnits=deg  RotationStandardAxis=+Z  RotationAngle=0.0  RotationArbitraryAxis=[0 0 1]  FollAlignAxisA=+X  BaseAlignAxisA=+Y  FollAlignAxisB=+Y  BaseAlignAxisB=+Z  RotationSequenceAxes=FollowerAxes  RotationSequence=XYX  RotationSequenceAngles=[0 0 0]  RotationSequenceAnglesUnits=deg  RotationMatrix=[1 0 0; 0 1 0; 0 0 1]  Quaternion=[1 0 0 0]
  T3 : sm_lib/Frames and Transforms/Rigid Transform  TranslationMethod=Cartesian  TranslationStandardOffset=0  TranslationStandardOffsetUnits=m  TranslationStandardAxis=+Z  TranslationCartesianOffset=[0 0 -3]  TranslationCartesianOffsetUnits=m  TranslationROffset=0  TranslationROffsetUnits=m  TranslationZOffset=0  TranslationZOffsetUnits=m  TranslationThetaOffset=0  TranslationThetaOffsetUnits=deg  RotationMethod=None  RotationAngleUnits=deg  RotationStandardAxis=+Z  RotationAngle=0.0  RotationArbitraryAxis=[0 0 1]  FollAlignAxisA=+X  BaseAlignAxisA=+Y  FollAlignAxisB=+Y  BaseAlignAxisB=+Z  RotationSequenceAxes=FollowerAxes  RotationSequence=XYX  RotationSequenceAngles=[0 0 0]  RotationSequenceAnglesUnits=deg  RotationMatrix=[1 0 0; 0 1 0; 0 0 1]  Quaternion=[1 0 0 0]
  T4 : sm_lib/Frames and Transforms/Rigid Transform  TranslationMethod=Cartesian  TranslationStandardOffset=0  TranslationStandardOffsetUnits=m  TranslationStandardAxis=+Z  TranslationCartesianOffset=[0 -2 0]  TranslationCartesianOffsetUnits=m  TranslationROffset=0  TranslationROffsetUnits=m  TranslationZOffset=0  TranslationZOffsetUnits=m  TranslationThetaOffset=0  TranslationThetaOffsetUnits=deg  RotationMethod=None  RotationAngleUnits=deg  RotationStandardAxis=+Z  RotationAngle=0.0  RotationArbitraryAxis=[0 0 1]  FollAlignAxisA=+X  BaseAlignAxisA=+Y  FollAlignAxisB=+Y  BaseAlignAxisB=+Z  RotationSequenceAxes=FollowerAxes  RotationSequence=XYX  RotationSequenceAngles=[0 0 0]  RotationSequenceAnglesUnits=deg  RotationMatrix=[1 0 0; 0 1 0; 0 0 1]  Quaternion=[1 0 0 0]
  T5 : sm_lib/Frames and Transforms/Rigid Transform  TranslationMethod=Cartesian  TranslationStandardOffset=0  TranslationStandardOffsetUnits=m  TranslationStandardAxis=+Z  TranslationCartesianOffset=[0 -2 0]  TranslationCartesianOffsetUnits=m  TranslationROffset=0  TranslationROffsetUnits=m  TranslationZOffset=0  TranslationZOffsetUnits=m  TranslationThetaOffset=0  TranslationThetaOffsetUnits=deg  RotationMethod=None  RotationAngleUnits=deg  RotationStandardAxis=+Z  RotationAngle=0.0  RotationArbitraryAxis=[0 0 1]  FollAlignAxisA=+X  BaseAlignAxisA=+Y  FollAlignAxisB=+Y  BaseAlignAxisB=+Z  RotationSequenceAxes=FollowerAxes  RotationSequence=XYX  RotationSequenceAngles=[0 0 0]  RotationSequenceAnglesUnits=deg  RotationMatrix=[1 0 0; 0 1 0; 0 0 1]  Quaternion=[1 0 0 0]
  T6 : sm_lib/Frames and Transforms/Rigid Transform  TranslationMethod=Cartesian  TranslationStandardOffset=0  TranslationStandardOffsetUnits=m  TranslationStandardAxis=+Z  TranslationCartesianOffset=[0 0 -3]  TranslationCartesianOffsetUnits=m  TranslationROffset=0  TranslationROffsetUnits=m  TranslationZOffset=0  TranslationZOffsetUnits=m  TranslationThetaOffset=0  TranslationThetaOffsetUnits=deg  RotationMethod=None  RotationAngleUnits=deg  RotationStandardAxis=+Z  RotationAngle=0.0  RotationArbitraryAxis=[0 0 1]  FollAlignAxisA=+X  BaseAlignAxisA=+Y  FollAlignAxisB=+Y  BaseAlignAxisB=+Z  RotationSequenceAxes=FollowerAxes  RotationSequence=XYX  RotationSequenceAngles=[0 0 0]  RotationSequenceAnglesUnits=deg  RotationMatrix=[1 0 0; 0 1 0; 0 0 1]  Quaternion=[1 0 0 0]
  T7 : sm_lib/Frames and Transforms/Rigid Transform  TranslationMethod=Cartesian  TranslationStandardOffset=0  TranslationStandardOffsetUnits=m  TranslationStandardAxis=+Z  TranslationCartesianOffset=[0 -3 0]  TranslationCartesianOffsetUnits=m  TranslationROffset=0  TranslationROffsetUnits=m  TranslationZOffset=0  TranslationZOffsetUnits=m  TranslationThetaOffset=0  TranslationThetaOffsetUnits=deg  RotationMethod=None  RotationAngleUnits=deg  RotationStandardAxis=+Z  RotationAngle=0.0  RotationArbitraryAxis=[0 0 1]  FollAlignAxisA=+X  BaseAlignAxisA=+Y  FollAlignAxisB=+Y  BaseAlignAxisB=+Z  RotationSequenceAxes=FollowerAxes  RotationSequence=XYX  RotationSequenceAngles=[0 0 0]  RotationSequenceAnglesUnits=deg  RotationMatrix=[1 0 0; 0 1 0; 0 0 1]  Quaternion=[1 0 0 0]
  T8 : sm_lib/Frames and Transforms/Rigid Transform  TranslationMethod=Cartesian  TranslationStandardOffset=0  TranslationStandardOffsetUnits=m  TranslationStandardAxis=+Z  TranslationCartesianOffset=[-2.5 0 0]  TranslationCartesianOffsetUnits=m  TranslationROffset=0  TranslationROffsetUnits=m  TranslationZOffset=0  TranslationZOffsetUnits=m  TranslationThetaOffset=0  TranslationThetaOffsetUnits=deg  RotationMethod=None  RotationAngleUnits=deg  RotationStandardAxis=+Z  RotationAngle=0.0  RotationArbitraryAxis=[0 0 1]  FollAlignAxisA=+X  BaseAlignAxisA=+Y  FollAlignAxisB=+Y  BaseAlignAxisB=+Z  RotationSequenceAxes=FollowerAxes  RotationSequence=XYX  RotationSequenceAngles=[0 0 0]  RotationSequenceAnglesUnits=deg  RotationMatrix=[1 0 0; 0 1 0; 0 0 1]  Quaternion=[1 0 0 0]
  T9 : sm_lib/Frames and Transforms/Rigid Transform  TranslationMethod=Cartesian  TranslationStandardOffset=0  TranslationStandardOffsetUnits=m  TranslationStandardAxis=+Z  TranslationCartesianOffset=[0 0 -2.5]  TranslationCartesianOffsetUnits=m  TranslationROffset=0  TranslationROffsetUnits=m  TranslationZOffset=0  TranslationZOffsetUnits=m  TranslationThetaOffset=0  TranslationThetaOffsetUnits=deg  RotationMethod=None  RotationAngleUnits=deg  RotationStandardAxis=+Z  RotationAngle=0.0  RotationArbitraryAxis=[0 0 1]  FollAlignAxisA=+X  BaseAlignAxisA=+Y  FollAlignAxisB=+Y  BaseAlignAxisB=+Z  RotationSequenceAxes=FollowerAxes  RotationSequence=XYX  RotationSequenceAngles=[0 0 0]  RotationSequenceAnglesUnits=deg  RotationMatrix=[1 0 0; 0 1 0; 0 0 1]  Quaternion=[1 0 0 0]
  Top : sm_lib/Frames and Transforms/Reference Frame
  World : sm_lib/Frames and Transforms/World Frame
  CoM : PMIOPort  Side=Right
  connections:
  T1/LConn1 -- T7/LConn1 -- SPH1/LConn1 -- CoM/RConn1 -- T6/LConn1
  Behind/RConn1 -- T3/RConn1 -- T2/LConn1 -- T1/RConn1
  BehindUP/RConn1 -- T2/RConn1 -- T5/RConn1 -- T4/LConn1
  T3/LConn1 -- BehindDown/RConn1
  BehindUPLeft/RConn1 -- T4/RConn1
  T5/LConn1 -- BehindUPRight/RConn1
  Top/RConn1 -- T6/RConn1
  Side/RConn1 -- T7/RConn1
  SPH1/RConn1 -- T8/LConn1 -- C1/LConn1 -- Negligible Mass/RConn1
  C1/RConn1 -- World/RConn1
  T9/LConn1 -- T8/RConn1
  T10/LConn1 -- T9/RConn1
  ISO/RConn1 -- T10/RConn1

== system AUV_Multi_MPC/AUV/Muiltibody/Hydro Forces & Moments ==
  Bus Element In : Inport  PortName=HydroForces  Element=Buoyancy.BForceZ
  Bus Element In1 : Inport  PortName=HydroForces  Element=LiftNDrag.LDForcesXYZ
  Bus Element In2 : Inport  PortName=HydroForces  Element=LiftNDrag.LDMomentsXYZ
  Bus Element In3 : Inport  PortName=HydroForces  Element=AddedMass.AMForcesXYZ
  Bus Element In4 : Inport  PortName=HydroForces  Element=AddedMass.AMMomentsXYZ
  Bus Element In5 : Inport  PortName=HydroForces  Element=AddedMass.CMomentsXYZ
  Bus Element In6 : Inport  PortName=HydroForces  Element=AddedMass.CForcesXYZ
  Added Mass Coriolis : Subsystem
  Added Mass Forces : Subsystem
  Buoyancy Force : Subsystem
  Lift and Drag Forces : Subsystem
  CoM : PMIOPort  Side=Right
  CoB : PMIOPort  Port=2  Side=Right
  wires:
  Bus Element In/1 -> Buoyancy Force/1(B)
  Bus Element In1/1 -> Lift and Drag Forces/1(Fxyz)
  Bus Element In2/1 -> Lift and Drag Forces/2(Mxyz)
  Bus Element In3/1 -> Added Mass Forces/1(Fxyz)
  Bus Element In4/1 -> Added Mass Forces/2(Mxyz)
  Bus Element In5/1 -> Added Mass Coriolis/2(Mxyz)
  Bus Element In6/1 -> Added Mass Coriolis/1(Fxyz)
  connections:
  CoB/RConn1 -- Buoyancy Force/RConn1
  Lift and Drag Forces/RConn1 -- Added Mass Coriolis/RConn1 -- Added Mass Forces/RConn1 -- CoM/RConn1

== system AUV_Multi_MPC/AUV/Muiltibody/World ==
  Mechanism Configuration : sm_lib/Utilities/Mechanism Configuration  UniformGravity=Constant  GravityVector=[0 0 Environment.gravity]  GravityVectorUnits=m/s^2  LinearizationDelta=0.001  JointModeTransitionNonlinearIterations=2
  Sea Floor : Subsystem
  Solver Configuration : nesl_utility/Solver Configuration  PhysicalDomain=network_engine_domain  SubClassName=solver  LeftPortType=input  RightPortType=generic  Tones=[]  Harmonics=[]  SimulateNoise=off  Profile=off  UseLocalSampling=off  EnableSwitchedLinearOptims=on  FrequencyDomain=off  UseCCode=off  RelTol=0.001  AbsTol=1e-06  MinStep=1e-09  ToWorkspace=off  RevertToSquareIcSolve=off  NumHomotopyIterations=100  PhasorMode=off  PhasorModeNumHarmonics=1  ConsistencySolver=NEWTON_FTOL  IndexReductionMethod=DerivativeReplacement  DoDC=off  ResidualTolerance=1e-09  ConsistencyTolSource=GLOBAL  ConsistencyAbsTol=0.001  ConsistencyRelTol=0.001  ConsistencyTolFactor=0.001  UseLocalSolver=off  LocalSolverChoice=NE_BACKWARD_EULER_ADVANCER  ResolveIndetEquations=on  FunctionEvalNumThread=1  LocalSolverSampleTime=0.001  DoFixedCost=off  MaxNonlinIter=3  MaxModeIter=2  ComputeImpulses=off  ImpulseIterations=2  LinearAlgebra=Sparse  LinearAlgebraNumThread=0  EquationFormulation=NE_TIME_EF  DelaysMemoryBudget=1024  AutomaticFiltering=on  FilteringTimeConstant=0.001  PartitionStorageMethod=AS_NEEDED  PartitionMemoryBudget=1024  PartitionMethod=FAST
  World Frame --> e NED : sm_lib/Frames and Transforms/World Frame
  W : PMIOPort  Side=Right
  connections:
  World Frame --> e NED/RConn1 -- W/RConn1 -- Sea Floor/LConn1 -- Mechanism Configuration/RConn1 -- Solver Configuration/RConn1

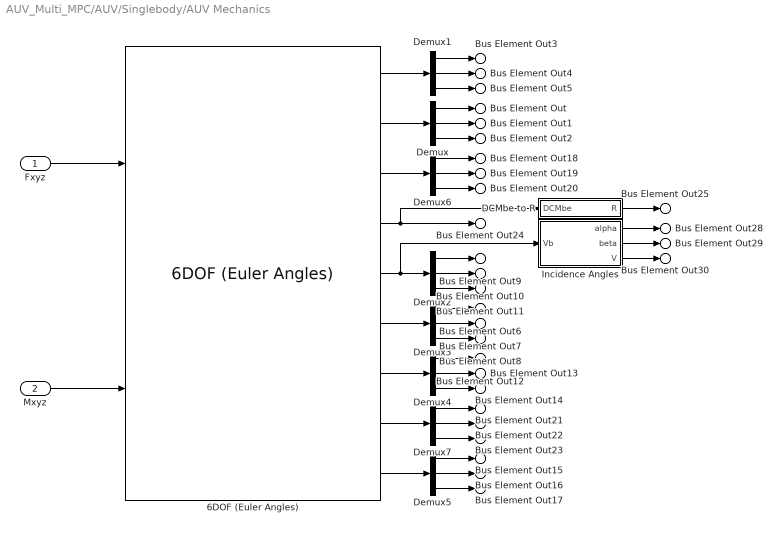
== system AUV_Multi_MPC/AUV/Singlebody/AUV Mechanics ==
  Fxyz : Inport
  Mxyz : Inport  Port=2
  6DOF (Euler Angles) : shared6dof/6DOF (Euler Angles)  units=Metric (MKS)  mtype=Fixed  rep=Euler Angles  xme_0=Vehicle.InitCond.position  Vm_0=Vehicle.InitCond.velocity  eul_0=Vehicle.InitCond.EulerXYZrad  pm_0=Vehicle.InitCond.rotrates  mass_0=Vehicle.Body.Full.mass  mass_e=0.5  mass_f=2.0  inertia=Vehicle.Body.Full.Inertia  inertia_e=eye(3)  inertia_f=2*eye(3)  k_quat=1.0  vre_flag=on  abi_flag=on  aMode=0  xme_statename=''  Vm_statename=''  eul_statename=''  quat_statename=''  pm_statename=''  mass_statename=''
  DCMbe to R : Subsystem
  Demux{,1..7} (8 alike) : Demux  Outputs=3
  Incidence Angles : Subsystem
  Bus Element Out : Outport  PortName=CoM  Element=World.Xe.X
  Bus Element Out1 : Outport  PortName=CoM  Element=World.Xe.Y
  Bus Element Out2 : Outport  PortName=CoM  Element=World.Xe.Z
  Bus Element Out3 : Outport  PortName=CoM  Element=World.Ve.Vx
  Bus Element Out4 : Outport  PortName=CoM  Element=World.Ve.Vy
  Bus Element Out5 : Outport  PortName=CoM  Element=World.Ve.Vz
  Bus Element Out25 : Outport  PortName=CoM  Element=World.R
  Bus Element Out6 : Outport  PortName=CoM  Element=Body.wb.p
  Bus Element Out7 : Outport  PortName=CoM  Element=Body.wb.q
  Bus Element Out8 : Outport  PortName=CoM  Element=Body.wb.r
  Bus Element Out9 : Outport  PortName=CoM  Element=Body.Vb.u
  Bus Element Out10 : Outport  PortName=CoM  Element=Body.Vb.v
  Bus Element Out11 : Outport  PortName=CoM  Element=Body.Vb.w
  Bus Element Out12 : Outport  PortName=CoM  Element=Body.dwbdt.pdot
  Bus Element Out13 : Outport  PortName=CoM  Element=Body.dwbdt.qdot
  Bus Element Out14 : Outport  PortName=CoM  Element=Body.dwbdt.rdot
  Bus Element Out15 : Outport  PortName=CoM  Element=Body.Abe.ax
  Bus Element Out16 : Outport  PortName=CoM  Element=Body.Abe.ay
  Bus Element Out17 : Outport  PortName=CoM  Element=Body.Abe.az
  Bus Element Out18 : Outport  PortName=CoM  Element=Derived.Euler.phi
  Bus Element Out19 : Outport  PortName=CoM  Element=Derived.Euler.theta
  Bus Element Out20 : Outport  PortName=CoM  Element=Derived.Euler.psi
  Bus Element Out21 : Outport  PortName=CoM  Element=Derived.Body.Abb.Abbx
  Bus Element Out22 : Outport  PortName=CoM  Element=Derived.Body.Abb.Abby
  Bus Element Out23 : Outport  PortName=CoM  Element=Derived.Body.Abb.Abbz
  Bus Element Out28 : Outport  PortName=CoM  Element=Derived.Body.Incidences.alpha
  Bus Element Out29 : Outport  PortName=CoM  Element=Derived.Body.Incidences.beta
  Bus Element Out30 : Outport  PortName=CoM  Element=Derived.Body.V
  Bus Element Out24 : Outport  PortName=CoM  Element=Derived.World.DCMbe
  wires:
  Fxyz/1 -> 6DOF (Euler Angles)/1
  6DOF (Euler Angles)/2 -> Demux/1
  Mxyz/1 -> 6DOF (Euler Angles)/2
  Demux/2 -> Bus Element Out1/1
  Demux/1 -> Bus Element Out/1
  Demux/3 -> Bus Element Out2/1
  6DOF (Euler Angles)/1 -> Demux1/1
  Demux1/1 -> Bus Element Out3/1
  Demux1/2 -> Bus Element Out4/1
  Demux1/3 -> Bus Element Out5/1
  6DOF (Euler Angles)/5 -> Demux2/1, Incidence Angles/1(Vb)
  6DOF (Euler Angles)/6 -> Demux3/1
  Demux3/1 -> Bus Element Out6/1
  Demux3/2 -> Bus Element Out7/1
  Demux3/3 -> Bus Element Out8/1
  Demux2/1 -> Bus Element Out9/1
  Demux2/2 -> Bus Element Out10/1
  Demux2/3 -> Bus Element Out11/1
  6DOF (Euler Angles)/7 -> Demux4/1
  Demux4/1 -> Bus Element Out12/1
  Demux4/2 -> Bus Element Out13/1
  Demux4/3 -> Bus Element Out14/1
  6DOF (Euler Angles)/9 -> Demux5/1
  Demux5/1 -> Bus Element Out15/1
  Demux5/2 -> Bus Element Out16/1
  Demux5/3 -> Bus Element Out17/1
  6DOF (Euler Angles)/3 -> Demux6/1
  Demux6/1 -> Bus Element Out18/1
  Demux6/2 -> Bus Element Out19/1
  Demux6/3 -> Bus Element Out20/1
  6DOF (Euler Angles)/8 -> Demux7/1
  Demux7/1 -> Bus Element Out21/1
  Demux7/2 -> Bus Element Out22/1
  Demux7/3 -> Bus Element Out23/1
  6DOF (Euler Angles)/4 -> Bus Element Out24/1, DCMbe to R/1(DCMbe)
  Incidence Angles/1(alpha) -> Bus Element Out28/1
  Incidence Angles/2(beta) -> Bus Element Out29/1
  Incidence Angles/3(V) -> Bus Element Out30/1
  DCMbe to R/1(R) -> Bus Element Out25/1

== system AUV_Multi_MPC/AUV/Singlebody/Hydro Forces & Moments ==
  Bus Element In : Inport  PortName=HydroForces  Element=Buoyancy.BForceZ
  Bus Element In1 : Inport  PortName=HydroForces  Element=Weight.WForceZ
  Bus Element In3 : Inport  PortName=HydroForces  Element=AddedMass.AMForcesXYZ
  Bus Element In4 : Inport  PortName=HydroForces  Element=AddedMass.AMMomentsXYZ
  Bus Element In5 : Inport  PortName=HydroForces  Element=AddedMass.CForcesXYZ
  Bus Element In6 : Inport  PortName=HydroForces  Element=AddedMass.CMomentsXYZ
  Bus Element In7 : Inport  PortName=HydroForces  Element=LiftNDrag.LDForcesXYZ
  Bus Element In8 : Inport  PortName=HydroForces  Element=LiftNDrag.LDMomentsXYZ
  Bus Element In2 : Inport  Port=2  PortName=CoM  Element=Derived.World.DCMbe
  Added Mass Forces : Subsystem
  Hydrostatic Forces : Subsystem
  Lift and Drag Forces : Subsystem
  Sum : Sum  Inputs=+++
  Sum1 : Sum  Inputs=+++
  Fxyz : Outport
  Mxyz : Outport  Port=2
  wires:
  Bus Element In2/1 -> Hydrostatic Forces/1(DCM)
  Bus Element In/1 -> Hydrostatic Forces/2(Bz)
  Bus Element In1/1 -> Hydrostatic Forces/3(Wz)
  Bus Element In3/1 -> Added Mass Forces/1(AMFxyz)
  Bus Element In4/1 -> Added Mass Forces/2(AMMxyz)
  Bus Element In5/1 -> Added Mass Forces/3(AMCFxyz)
  Bus Element In6/1 -> Added Mass Forces/4(AMCMxyz)
  Bus Element In7/1 -> Lift and Drag Forces/1(LDFxyz)
  Bus Element In8/1 -> Lift and Drag Forces/2(LDMxyz)
  Lift and Drag Forces/1(Fxyz) -> Sum/2
  Sum/1 -> Fxyz/1
  Hydrostatic Forces/1(Fxyz) -> Sum/1
  Added Mass Forces/1(Fxyz) -> Sum/3
  Sum1/1 -> Mxyz/1
  Lift and Drag Forces/2(Mxyz) -> Sum1/2
  Hydrostatic Forces/2(Mxyz) -> Sum1/1
  Added Mass Forces/2(Mxyz) -> Sum1/3

== system AUV_Multi_MPC/AUV/Singlebody/Propellers & Thrusters ==
  Bus Element In : Inport  PortName=Actuators  Element=Propellers.PPf
  Bus Element In1 : Inport  PortName=Actuators  Element=Propellers.SPf
  Bus Element In2 : Inport  PortName=Actuators  Element=Thrusters.BHTf
  Bus Element In3 : Inport  PortName=Actuators  Element=Thrusters.BVTf
  Bus Element In4 : Inport  PortName=Actuators  Element=Thrusters.SHTf
  Bus Element In5 : Inport  PortName=Actuators  Element=Thrusters.SVTf
  Horizontal Tunnel Thrusters : Subsystem
  Main Propellers : Subsystem
  Sum : Sum  Inputs=+++
  Sum1 : Sum  Inputs=+++
  Vertical Tunnel Thrusters : Subsystem
  Fxyz : Outport
  Mxyz : Outport  Port=2
  wires:
  Bus Element In1/1 -> Main Propellers/1(SPf)
  Bus Element In/1 -> Main Propellers/2(PPf)
  Bus Element In3/1 -> Vertical Tunnel Thrusters/1(BVTf)
  Bus Element In5/1 -> Vertical Tunnel Thrusters/2(SVTf)
  Bus Element In2/1 -> Horizontal Tunnel Thrusters/1(BHTf)
  Bus Element In4/1 -> Horizontal Tunnel Thrusters/2(SHTf)
  Horizontal Tunnel Thrusters/1(Fxyz) -> Sum/2
  Sum/1 -> Fxyz/1
  Main Propellers/1(Fxyz) -> Sum/1
  Vertical Tunnel Thrusters/1(Fxyz) -> Sum/3
  Sum1/1 -> Mxyz/1
  Horizontal Tunnel Thrusters/2(Mxyz) -> Sum1/2
  Main Propellers/2(Mxyz) -> Sum1/1
  Vertical Tunnel Thrusters/2(Mxyz) -> Sum1/3

== system AUV_Multi_MPC/Dive Controls/Thrust Controls/Adaptive MPC control surge ==
  Feedback : Inport
  Reference : Inport  Port=2
  Adaptive MPC Controller : mpclib/Adaptive MPC Controller  SCDEnableBlockLinearizationSpecification=on  mpcobj=mpc1  enable_value=0  updateMPCinCallerWorkspace=on  md_inport=off  mv_inport=off  uref_inport=off  return_cost=off  return_mvseq=off  return_qpstatus=off  return_xseq=off  return_state=off  return_ovseq=off  state_inport=off  isltv_plant=off  umin_inport=off  umax_inport=off  ymin_inport=off  ymax_inport=off  cc_inport=off  ywt_inport=off  uwt_inport=off  duwt_inport=off  rhoeps_inport=off  pm_inport=off  MaximumP=10  HorizonChoice=FixedHorizon  BlockDataType=double  SampleTimeInherited=off  switch_inport=off
  Bus Creator : BusCreator  Inputs=8
  MATLAB Function : MATLAB Function  TreatAsAtomicUnit=on
  Scope : Scope  NumInputPorts=2
  Scope1 : Scope
  PPfcmd : Outport
  SPfcmd : Outport  Port=2
  wires:
  Bus Creator/1 -> Adaptive MPC Controller/1
  MATLAB Function/7(DX) -> Bus Creator/7
  MATLAB Function/4(D) -> Bus Creator/4
  MATLAB Function/6(Y) -> Bus Creator/6
  MATLAB Function/2(B) -> Bus Creator/2
  MATLAB Function/3(C) -> Bus Creator/3
  MATLAB Function/1(A) -> Bus Creator/1
  Reference/1 -> Scope/2, Adaptive MPC Controller/3
  MATLAB Function/8(U) -> Bus Creator/8
  Feedback/1 -> Scope/1, Adaptive MPC Controller/2, MATLAB Function/1(x)
  Adaptive MPC Controller/1 -> SPfcmd/1, MATLAB Function/2(u), PPfcmd/1, Scope1/1
  MATLAB Function/5(X) -> Bus Creator/5
